simulink model "nyquist_basic"  (Simulink 8.5)
settings: Solver=ode3  StartTime=0.0  StopTime=600  FixedStep=1e-3  RelTol=1e-3
settings Model: Creator=henrik  LastModifiedBy=hg35a  CovSFcnEnable=off
settings DataIOCC: SignalLoggingName=sigsOut
settings OptimizationCC: InitFltsAndDblsToZero=on
settings DebuggingCC: SaveWithParameterizedLinksMsg=none  SignalResolutionControl=TryResolveAllWithWarning  MultiTaskDSMMsg=warning  MultiTaskCondExecSysMsg=none  FcnCallInpInsideContextMsg=UseLocalSettings
settings HardwareCC: TargetUnknown=on
settings GRTTargetCC: TargetFcnLib=ansi_tfl_tmw.mat  ModelReferenceCompliant=off  MatFileLogging=off

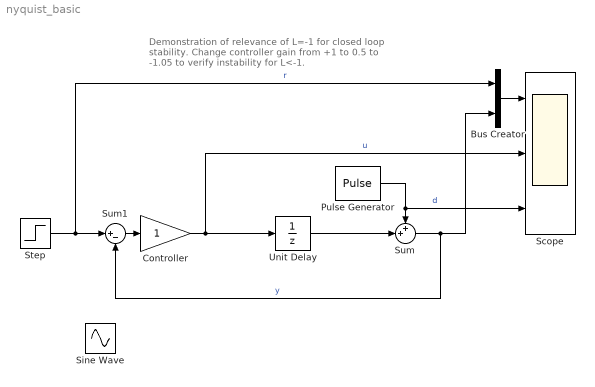
== system nyquist_basic ==
  note: Demonstration of relevance of L=-1
      | for closed loop stability.
      | Change controller gain from +1 to 0.5 to -1.05
      | to verify instability for L<-1.
  Bus Creator : BusCreator  Inputs=2
  Controller : Gain
  Pulse Generator : DiscretePulseGenerator  PulseType=Time based  Amplitude=0  Period=60  PulseWidth=50  PhaseDelay=30
  Scope : Scope  NumInputPorts=3
      settings: ShowLegends=on  YMin=-100~-100~-1  YMax=10~0~1
  Sine Wave : Sin  SampleTime=0
  Step : Step  SampleTime=0
  Sum : Sum  Inputs=++|  SaturateOnIntegerOverflow=on
  Sum1 : Sum  Inputs=|+-  SaturateOnIntegerOverflow=on
  Unit Delay : UnitDelay  SampleTime=-1
  wires:
  Controller/1 -> Unit Delay/1, Scope/2  "u"
  Pulse Generator/1 -> Sum/1, Scope/3  "d"
  Step/1 -> Bus Creator/1, Sum1/1  "r"
  Bus Creator/1 -> Scope/1
  Sum/1 -> Bus Creator/2, Sum1/2  "y"
  Sum1/1 -> Controller/1
  Unit Delay/1 -> Sum/2
